simulink model "practico_2_3"  (R2024b)
settings: Solver=VariableStepAuto  StartTime=0.0  StopTime=600  RelTol=1e-3
values from neighbouring files (symbols this model uses):
  F_in = 0.0035    [p2_code.m]
  F_out_sin_k = a_tub*sqrt(2*g)    [p2_code.m]
  h_list = [0.2, 0.4, 0.6, 0.8]    [p2_code.m]
  k_list = zeros(1, length(h_list))    [p2_code.m]
  r_0 = 0.05    [p2_code.m]
  theta = 60    [p2_code.m]
undefined symbols (not defined in the file or in its folder): A, B, C, D
settings Model: Creator=trulscarlson  LastModifiedBy=trulscarlson
settings DebuggingCC: UnconnectedInputMsg=warning  UnconnectedOutputMsg=warning  UnconnectedLineMsg=warning
settings ModelReferenceCC: EnableRefExpFcnMdlSchedulingChecks=on
settings RTWCC: GPUComputeCapability=3.5  DLArmComputeVersion=19.05

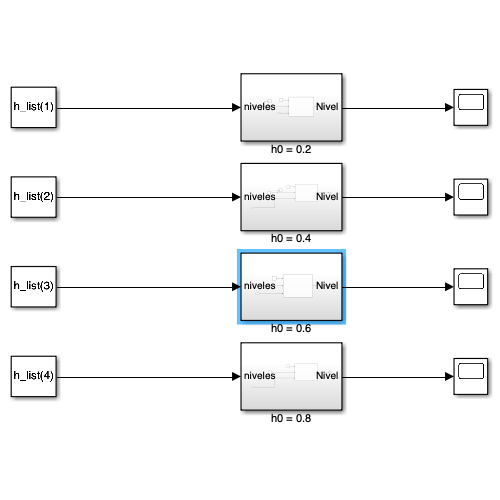
[thumbnail: Simulink's stored preview of the top-level diagram]
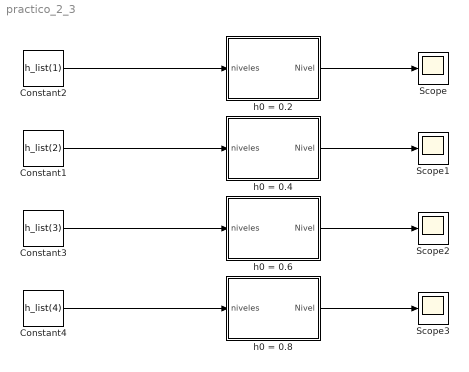
== system practico_2_3 ==
  Constant1 : Constant  Value=h_list(2)
  Constant2 : Constant  Value=h_list(1)
  Constant3 : Constant  Value=h_list(3)
  Constant4 : Constant  Value=h_list(4)
  Scope{,1..3} (4 alike) : Scope
  h0 = 0.2 : Subsystem
  h0 = 0.4 : Subsystem
  h0 = 0.6 : Subsystem
  h0 = 0.8 : Subsystem
  wires:
  Constant4/1 -> h0 = 0.8/1(niveles)
  h0 = 0.2/1(Nivel) -> Scope/1
  Constant2/1 -> h0 = 0.2/1(niveles)
  Constant1/1 -> h0 = 0.4/1(niveles)
  h0 = 0.4/1(Nivel) -> Scope1/1
  h0 = 0.8/1(Nivel) -> Scope3/1
  Constant3/1 -> h0 = 0.6/1(niveles)
  h0 = 0.6/1(Nivel) -> Scope2/1

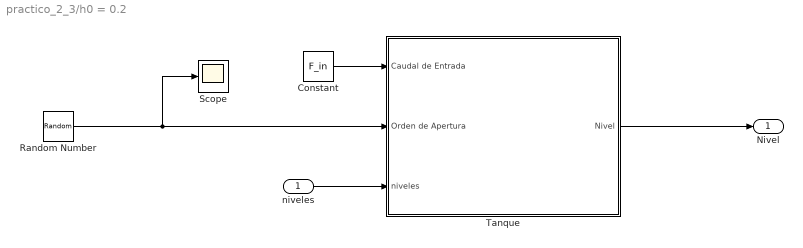
== system practico_2_3/h0 = 0.2 ==
  niveles : Inport
  Constant : Constant  Value=F_in
  Random Number : RandomNumber  Mean=k_list(1)  Variance=0.001  SampleTime=0.2
  Scope : Scope
  Tanque : Subsystem
  Nivel : Outport
  wires:
  niveles/1 -> Tanque/3(niveles)
  Constant/1 -> Tanque/1(Caudal de Entrada)
  Tanque/1(Nivel) -> Nivel/1
  Random Number/1 -> Scope/1, Tanque/2(Orden de Apertura)

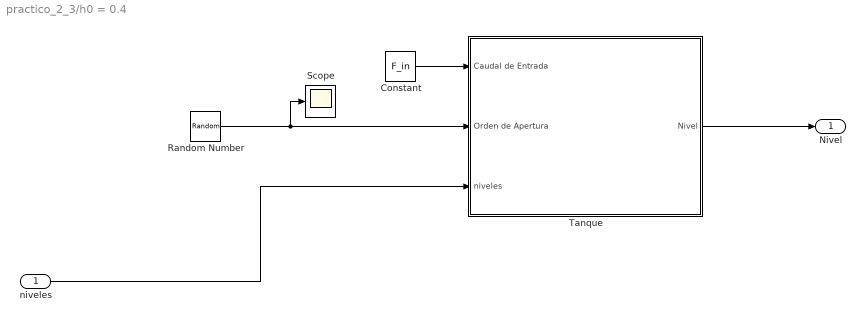
== system practico_2_3/h0 = 0.4 ==
  niveles : Inport
  Constant : Constant  Value=F_in
  Random Number : RandomNumber  Mean=k_list(2)  Variance=0.001  SampleTime=0.2
  Scope : Scope
  Tanque : Subsystem
  Nivel : Outport
  wires:
  niveles/1 -> Tanque/3(niveles)
  Constant/1 -> Tanque/1(Caudal de Entrada)
  Tanque/1(Nivel) -> Nivel/1
  Random Number/1 -> Scope/1, Tanque/2(Orden de Apertura)

== system practico_2_3/h0 = 0.6 ==
  niveles : Inport
  Constant : Constant  Value=F_in
  Random Number : RandomNumber  Mean=k_list(3)  Variance=0.001  SampleTime=0.2
  Tanque : Subsystem
  Nivel : Outport
  wires:
  niveles/1 -> Tanque/3(niveles)
  Constant/1 -> Tanque/1(Caudal de Entrada)
  Tanque/1(Nivel) -> Nivel/1
  Random Number/1 -> Tanque/2(Orden de Apertura)

== system practico_2_3/h0 = 0.8 ==
  niveles : Inport
  Constant : Constant  Value=F_in
  Random Number : RandomNumber  Mean=k_list(4)  Variance=0.001  SampleTime=0.2
  Tanque : Subsystem
  Nivel : Outport
  wires:
  niveles/1 -> Tanque/3(niveles)
  Constant/1 -> Tanque/1(Caudal de Entrada)
  Tanque/1(Nivel) -> Nivel/1
  Random Number/1 -> Tanque/2(Orden de Apertura)

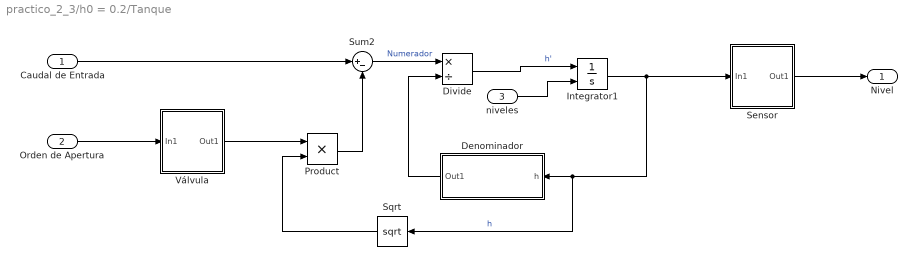
== system practico_2_3/h0 = 0.2/Tanque ==
  Caudal de Entrada : Inport
  Orden de Apertura : Inport  Port=2
  niveles : Inport  Port=3
  Denominador : Subsystem
  Divide : Product  Inputs=*/
  Integrator1 : Integrator  InitialConditionSource=external  InitialCondition=h_list(5)
  Product : Product
  Sensor : Subsystem
  Sqrt : Sqrt
  Sum2 : Sum  Inputs=|+-
  Válvula : Subsystem
  Nivel : Outport
  wires:
  Product/1 -> Sum2/2
  Divide/1 -> Integrator1/1  "h'"
  Denominador/1(Out1) -> Divide/2
  Integrator1/1 -> Sensor/1(In1), Sqrt/1, Denominador/1(h)  "h"
  Sum2/1 -> Divide/1  "Numerador"
  Sqrt/1 -> Product/2
  Caudal de Entrada/1 -> Sum2/1
  Orden de Apertura/1 -> Válvula/1(In1)
  Válvula/1(Out1) -> Product/1
  niveles/1 -> Integrator1/2
  Sensor/1(Out1) -> Nivel/1

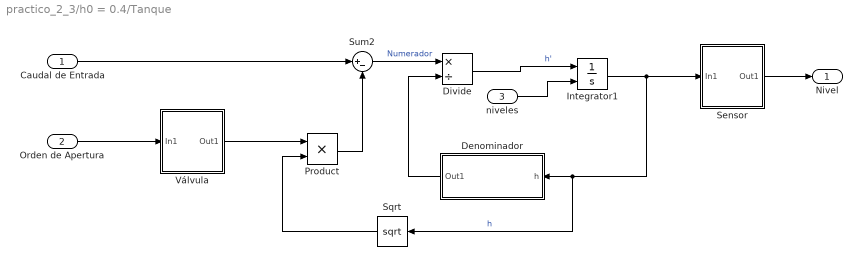
== system practico_2_3/h0 = 0.4/Tanque ==
  Caudal de Entrada : Inport
  Orden de Apertura : Inport  Port=2
  niveles : Inport  Port=3
  Denominador : Subsystem
  Divide : Product  Inputs=*/
  Integrator1 : Integrator  InitialConditionSource=external  InitialCondition=h_list(5)
  Product : Product
  Sensor : Subsystem
  Sqrt : Sqrt
  Sum2 : Sum  Inputs=|+-
  Válvula : Subsystem
  Nivel : Outport
  wires:
  Product/1 -> Sum2/2
  Divide/1 -> Integrator1/1  "h'"
  Denominador/1(Out1) -> Divide/2
  Integrator1/1 -> Sensor/1(In1), Sqrt/1, Denominador/1(h)  "h"
  Sum2/1 -> Divide/1  "Numerador"
  Sqrt/1 -> Product/2
  Caudal de Entrada/1 -> Sum2/1
  Orden de Apertura/1 -> Válvula/1(In1)
  Válvula/1(Out1) -> Product/1
  niveles/1 -> Integrator1/2
  Sensor/1(Out1) -> Nivel/1

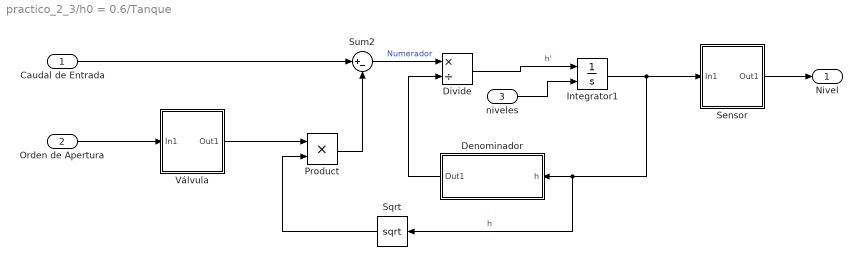
== system practico_2_3/h0 = 0.6/Tanque ==
  Caudal de Entrada : Inport
  Orden de Apertura : Inport  Port=2
  niveles : Inport  Port=3
  Denominador : Subsystem
  Divide : Product  Inputs=*/
  Integrator1 : Integrator  InitialConditionSource=external  InitialCondition=h_list(5)
  Product : Product
  Sensor : Subsystem
  Sqrt : Sqrt
  Sum2 : Sum  Inputs=|+-
  Válvula : Subsystem
  Nivel : Outport
  wires:
  Product/1 -> Sum2/2
  Divide/1 -> Integrator1/1  "h'"
  Denominador/1(Out1) -> Divide/2
  Integrator1/1 -> Sensor/1(In1), Sqrt/1, Denominador/1(h)  "h"
  Sum2/1 -> Divide/1  "Numerador"
  Sqrt/1 -> Product/2
  Caudal de Entrada/1 -> Sum2/1
  Orden de Apertura/1 -> Válvula/1(In1)
  Válvula/1(Out1) -> Product/1
  niveles/1 -> Integrator1/2
  Sensor/1(Out1) -> Nivel/1

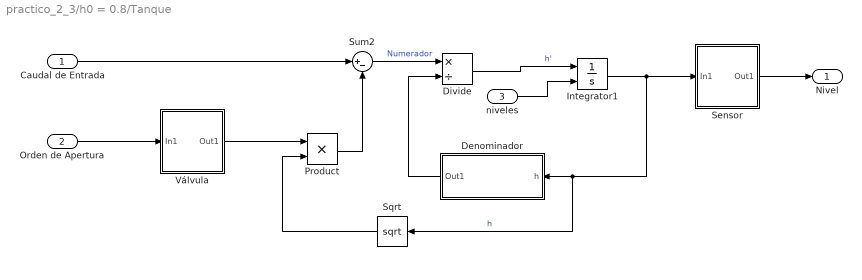
== system practico_2_3/h0 = 0.8/Tanque ==
  Caudal de Entrada : Inport
  Orden de Apertura : Inport  Port=2
  niveles : Inport  Port=3
  Denominador : Subsystem
  Divide : Product  Inputs=*/
  Integrator1 : Integrator  InitialConditionSource=external  InitialCondition=h_list(5)
  Product : Product
  Sensor : Subsystem
  Sqrt : Sqrt
  Sum2 : Sum  Inputs=|+-
  Válvula : Subsystem
  Nivel : Outport
  wires:
  Product/1 -> Sum2/2
  Divide/1 -> Integrator1/1  "h'"
  Denominador/1(Out1) -> Divide/2
  Integrator1/1 -> Sensor/1(In1), Sqrt/1, Denominador/1(h)  "h"
  Sum2/1 -> Divide/1  "Numerador"
  Sqrt/1 -> Product/2
  Caudal de Entrada/1 -> Sum2/1
  Orden de Apertura/1 -> Válvula/1(In1)
  Válvula/1(Out1) -> Product/1
  niveles/1 -> Integrator1/2
  Sensor/1(Out1) -> Nivel/1

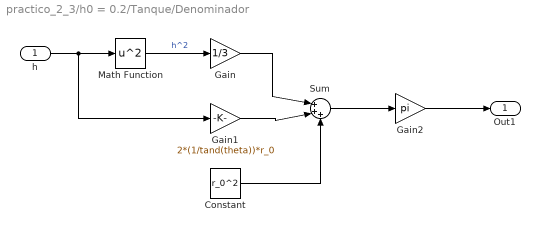
== system practico_2_3/h0 = 0.2/Tanque/Denominador ==
  h : Inport
  Constant : Constant  Value=r_0^2
  Gain : Gain  Gain=1/3
  Gain1 : Gain  Gain=2*(1/tand(theta))*r_0
  Gain2 : Gain  Gain=pi
  Math Function : Math  Operator=square
  Sum : Sum  Inputs=|+++
  Out1 : Outport
  wires:
  h/1 -> Gain1/1, Math Function/1
  Math Function/1 -> Gain/1  "h^2"
  Gain/1 -> Sum/1
  Gain1/1 -> Sum/2
  Constant/1 -> Sum/3
  Sum/1 -> Gain2/1
  Gain2/1 -> Out1/1

== system practico_2_3/h0 = 0.2/Tanque/Sensor ==
  In1 : Inport
  State-Space : StateSpace  A=A  B=B  C=C  D=D  InitialCondition=h_list(1)*10
  Out1 : Outport
  wires:
  In1/1 -> State-Space/1
  State-Space/1 -> Out1/1

== system practico_2_3/h0 = 0.2/Tanque/Válvula ==
  In1 : Inport
  Gain : Gain  Gain=F_out_sin_k
  State-Space : StateSpace  A=A  B=B  C=C  D=D  InitialCondition=k_list(1)*10
  Out1 : Outport
  wires:
  State-Space/1 -> Gain/1
  Gain/1 -> Out1/1
  In1/1 -> State-Space/1

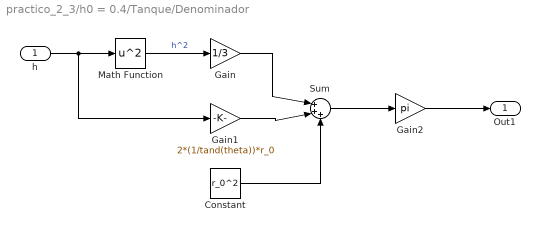
== system practico_2_3/h0 = 0.4/Tanque/Denominador ==
  h : Inport
  Constant : Constant  Value=r_0^2
  Gain : Gain  Gain=1/3
  Gain1 : Gain  Gain=2*(1/tand(theta))*r_0
  Gain2 : Gain  Gain=pi
  Math Function : Math  Operator=square
  Sum : Sum  Inputs=|+++
  Out1 : Outport
  wires:
  h/1 -> Gain1/1, Math Function/1
  Math Function/1 -> Gain/1  "h^2"
  Gain/1 -> Sum/1
  Gain1/1 -> Sum/2
  Constant/1 -> Sum/3
  Sum/1 -> Gain2/1
  Gain2/1 -> Out1/1

== system practico_2_3/h0 = 0.4/Tanque/Sensor ==
  In1 : Inport
  State-Space : StateSpace  A=A  B=B  C=C  D=D  InitialCondition=h_list(2)*10
  Out1 : Outport
  wires:
  In1/1 -> State-Space/1
  State-Space/1 -> Out1/1

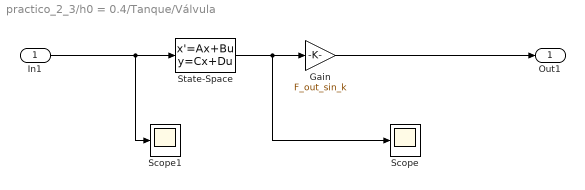
== system practico_2_3/h0 = 0.4/Tanque/Válvula ==
  In1 : Inport
  Gain : Gain  Gain=F_out_sin_k
  Scope : Scope
  Scope1 : Scope
  State-Space : StateSpace  A=A  B=B  C=C  D=D  InitialCondition=k_list(2)*10
  Out1 : Outport
  wires:
  State-Space/1 -> Gain/1, Scope/1
  Gain/1 -> Out1/1
  In1/1 -> Scope1/1, State-Space/1

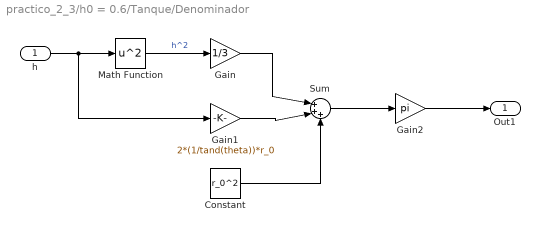
== system practico_2_3/h0 = 0.6/Tanque/Denominador ==
  h : Inport
  Constant : Constant  Value=r_0^2
  Gain : Gain  Gain=1/3
  Gain1 : Gain  Gain=2*(1/tand(theta))*r_0
  Gain2 : Gain  Gain=pi
  Math Function : Math  Operator=square
  Sum : Sum  Inputs=|+++
  Out1 : Outport
  wires:
  h/1 -> Gain1/1, Math Function/1
  Math Function/1 -> Gain/1  "h^2"
  Gain/1 -> Sum/1
  Gain1/1 -> Sum/2
  Constant/1 -> Sum/3
  Sum/1 -> Gain2/1
  Gain2/1 -> Out1/1

== system practico_2_3/h0 = 0.6/Tanque/Sensor ==
  In1 : Inport
  State-Space : StateSpace  A=A  B=B  C=C  D=D  InitialCondition=h_list(3)*10
  Out1 : Outport
  wires:
  In1/1 -> State-Space/1
  State-Space/1 -> Out1/1

== system practico_2_3/h0 = 0.6/Tanque/Válvula ==
  In1 : Inport
  Gain : Gain  Gain=F_out_sin_k
  Scope : Scope
  Scope1 : Scope
  State-Space : StateSpace  A=A  B=B  C=C  D=D  InitialCondition=k_list(3)*10
  Out1 : Outport
  wires:
  State-Space/1 -> Gain/1, Scope/1
  Gain/1 -> Out1/1
  In1/1 -> Scope1/1, State-Space/1

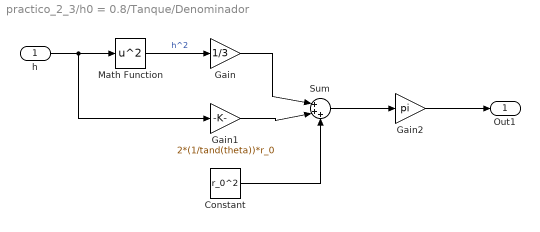
== system practico_2_3/h0 = 0.8/Tanque/Denominador ==
  h : Inport
  Constant : Constant  Value=r_0^2
  Gain : Gain  Gain=1/3
  Gain1 : Gain  Gain=2*(1/tand(theta))*r_0
  Gain2 : Gain  Gain=pi
  Math Function : Math  Operator=square
  Sum : Sum  Inputs=|+++
  Out1 : Outport
  wires:
  h/1 -> Gain1/1, Math Function/1
  Math Function/1 -> Gain/1  "h^2"
  Gain/1 -> Sum/1
  Gain1/1 -> Sum/2
  Constant/1 -> Sum/3
  Sum/1 -> Gain2/1
  Gain2/1 -> Out1/1

== system practico_2_3/h0 = 0.8/Tanque/Sensor ==
  In1 : Inport
  State-Space : StateSpace  A=A  B=B  C=C  D=D  InitialCondition=h_list(4)*10
  Out1 : Outport
  wires:
  In1/1 -> State-Space/1
  State-Space/1 -> Out1/1

== system practico_2_3/h0 = 0.8/Tanque/Válvula ==
  In1 : Inport
  Gain : Gain  Gain=F_out_sin_k
  Scope : Scope
  Scope1 : Scope
  State-Space : StateSpace  A=A  B=B  C=C  D=D  InitialCondition=k_list(4)*10
  Out1 : Outport
  wires:
  State-Space/1 -> Gain/1, Scope/1
  Gain/1 -> Out1/1
  In1/1 -> Scope1/1, State-Space/1
